simulink subsystem "Controls"  (R2024b)
settings: Solver=VariableStepAuto  StartTime=0.0  StopTime=10.0  RelTol=1e-3
undefined symbols (not defined in the file): D1, DiscIntNeverNeededParam, lag, Tctrl, test_alpha, Ts, Yg
libraries: powerlib_extras x74, simulink x10
(part 2 of 7)

== system Controls/fault_trigger ==
  pulse : Inport
  set : Inport  Port=2
  Compare To Constant{1..4,6..7} (6 alike) : simulink/Logic and Bit Operations/Compare To Constant  relop=>=  const=0.5  OutDataTypeStr=uint8  ZeroCross=off
  Constant : Constant  Value=[0 0]
  Demux1 : Demux  Outputs=[7 1 7]
  Demux2 : Demux  Outputs=[1 3 3]
  Demux4 : Demux  Outputs=7
  Mux9 : Mux  Inputs=8
  Product{1..4,6..10} (9 alike) : Product  RndMeth=Zero
  Terminator : Terminator
  faultgen : Subsystem
  DCtrig : Outport
  fault : Outport  Port=2
  wires:
  faultgen/3(trig) -> DCtrig/1  "trigger sig"
  pulse/1 -> faultgen/5(pulse)
  faultgen/1(fault) -> Product9/2, Product8/2, Product7/2, Product4/2, Product3/2, Product2/2, Product1/2
  Constant/1 -> faultgen/4(pert_set)
  Demux2/2 -> faultgen/2(Tst_set)
  Demux2/1 -> faultgen/1(Tacq)
  Demux2/3 -> faultgen/3(Tdr_set)
  faultgen/2(pertb) -> Terminator/1
  Demux1/2 -> Mux9/8
  Demux1/1 -> Demux4/1
  set/1 -> Demux1/1
  Mux9/1 -> fault/1
  Product9/1 -> Product10/1
  Product10/1 -> Mux9/7  "inv_fault"
  Demux4/7 -> Product10/2, Compare To Constant7/1
  Compare To Constant7/1 -> Product9/1
  Demux4/6 -> Product6/2, Compare To Constant6/1
  Demux4/5 -> Product7/1
  Demux4/4 -> Compare To Constant4/1
  Demux4/3 -> Compare To Constant3/1
  Demux4/2 -> Compare To Constant2/1
  Demux4/1 -> Compare To Constant1/1
  Demux1/3 -> Demux2/1
  Product8/1 -> Product6/1
  Compare To Constant6/1 -> Product8/1
  Product7/1 -> Mux9/6  "Fault_ac"
  Product4/1 -> Mux9/4  "Fault_dc"
  Compare To Constant4/1 -> Product4/1
  Product3/1 -> Mux9/3  "gammastep"
  Compare To Constant3/1 -> Product3/1
  Product2/1 -> Mux9/2  "Vdstep"
  Compare To Constant2/1 -> Product2/1
  Product1/1 -> Mux9/1  "Idrefstep"
  Compare To Constant1/1 -> Product1/1
  Product6/1 -> Mux9/5  "rect_fault"

== system Controls/paraconv ==
  In1 : Inport
  Demux : Demux  Outputs=[2 2 2 ]
  Kp/Ki-Ki to Kp Ki1 : Subsystem
  Kp/Ki-Ki to Kp Ki2 : Subsystem
  Kp/Ki-Ki to Kp Ki3 : Subsystem
  Mux2 : Mux  Inputs=3
  Out1 : Outport
  wires:
  Demux/3 -> Kp/Ki-Ki to Kp Ki3/1(i)
  Demux/2 -> Kp/Ki-Ki to Kp Ki2/1(i)  "KinvG"
  Demux/1 -> Kp/Ki-Ki to Kp Ki1/1(i)  "KinvV"
  In1/1 -> Demux/1
  Mux2/1 -> Out1/1
  Kp/Ki-Ki to Kp Ki3/1(o) -> Mux2/3
  Kp/Ki-Ki to Kp Ki2/1(o) -> Mux2/2
  Kp/Ki-Ki to Kp Ki1/1(o) -> Mux2/1

== system Controls/Master Control/Informations ==
  note: At start-up, both converters are deblocked and ramped up to the minimum current allowed in steady-state
      | with an adjustable rate  and application time in the "Start/Stop & Ramping Unit" subsystem. After the
      | system stabilisation the current is ramped up to its final value  with an adjustable rate and execution time.
      | Before stopping the converters the current is ramped down to the minimum reference.
  note: DESCRIPTION
  note: The rectifier and inverter current reference are generated in the master control. The reference
      | should be equal in both converters to avoid the loss of the margin. The converter starting and stopping is
      | initiated and the current reference can be ramped up or down.  A current step can be added to the
      | current reference for testing purpose.
  note: INTRODUCTION
  note: Master Control
  note: For testing purpose,  a step can be activated and added to the reference current at both
      | converters.

== system Controls/Master Control/Start//Stop ==
  note: Ramping
      | (modified from SPS demo)
  note: Start/Stop & Ramping
  note: Start/Stop sequence
  start : Inport
  Discrete Bistable : powerlib_extras/Discrete  Control Blocks/Discrete Bistable  Priority=488689760  SPSpriority=Set  ic=0  Ts=dt
  Discrete Edge Detector1 : powerlib_extras/Discrete  Control Blocks/Discrete Edge Detector  model=Rising  ic=0  Ts=dt
  Discrete Edge Detector2 : powerlib_extras/Discrete  Control Blocks/Discrete Edge Detector  model=Rising  ic=0  Ts=dt
  Logical Operator1 : Logic  Operator=NOT  AllPortsSameDT=off
  Logical Operator3 : Logic  AllPortsSameDT=off
  Minimum ref : Constant  Value=Min_ref
  Relational Operator1 : RelationalOperator  Operator=<=  InputSameDT=off
  S1 : Subsystem  mask(RAMPING UNIT){Min_ref=Min_ref, SS_ramp=SS_ramp, F_up=F_up, up_slope=up_slope, T_up=T_up, F_down=F_down, down_slope=down_slope, T_down=T_down}
      mask prompts: Min_ref "Minimum Value (pu):"; SS_ramp "Start-Stop ramp (pu/s):"; F_up "Final Up Value (pu):"; up_slope "Up Slope (pu/s):"; T_up "Ramping Up Time (s):"; F_down "Final Down Value (pu):"; down_slope "Down Slope (pu/s):"; T_down "Ramping Down Time (s):"
      mask init:
      | T_up_final      =  T_up + (F_up - Min_ref)/up_slope;
      | T_down_final =   T_down + (F_down-F_up)/down_slope;
      | T_ramp  = [0, T_up, T_up_final,  T_down,  T_down_final, 9999]';
      | U_ramp = [0, 0, F_up-Min_ref,  F_up-Min_ref,  F_down- Min_ref,  F_down - Min_ref]';
      mask Display: disp('Ramping\n Unit')
  Unit Delay : UnitDelay  SampleTime=dt  HasFrameUpgradeWarning=on
  Id_ref_ramp : Outport
  "Stop " : Outport  Port=2
  wires:
  Logical Operator1/1 -> Logical Operator3/2
  start/1 -> Logical Operator1/1, S1/1(Start), Discrete Edge Detector1/1
  Discrete Edge Detector1/1 -> Discrete Bistable/1
  Relational Operator1/1 -> Logical Operator3/1
  Logical Operator3/1 -> Discrete Edge Detector2/1
  Unit Delay/1 -> Relational Operator1/1
  Minimum ref/1 -> Relational Operator1/2
  Discrete Bistable/2 -> "Stop "/1
  S1/1(Out1) -> Id_ref_ramp/1, Unit Delay/1
  Discrete Edge Detector2/1 -> Discrete Bistable/2

== system Controls/Pole 1 Inverter Control and Protection/12-pulse Firing Control ==
  alpha_ord (deg) : Inport
  Vabc (pu) : Inport  Port=2
  Block : Inport  Port=3
  Data Type Conversion : DataTypeConversion  OutDataTypeStr=double
  Mux1 : Mux  Inputs=6
  PLL : Subsystem
  Freq : Outport
  fpu_I : Outport  Port=2
  wires:
  PLL/3(Vc) -> Mux1/4
  PLL/2(Vb) -> Mux1/3
  PLL/1(Va) -> Mux1/2
  Mux1/1 -> fpu_I/1
  Data Type Conversion/1 -> Mux1/6
  Block/1 -> Data Type Conversion/1
  alpha_ord (deg)/1 -> Mux1/1
  PLL/4(Freq) -> Mux1/5, Freq/1
  Vabc (pu)/1 -> PLL/1(Vabc(pu))

== system Controls/Pole 1 Inverter Control and Protection/Gamma Measurement ==
  note: PU scaling is made
      | in the SS_
  note: PU scaling is made
      | in the SS_
  Vabc : Inport
  Freq : Inport  Port=2
  IthyY : Inport  Port=3
  IthyD : Inport  Port=4
  Discrete Gamma Measurement (D bridge) : powerlib_extras/Discrete  Control Blocks/Discrete Gamma Measurement  transfo_type=Yg / D1(lag)  f0=50  Ith_min=0.001  Interpolation=off  V_tol=0.01  Ts=Tctrl
  Discrete Gamma Measurement (Y bridge) : powerlib_extras/Discrete  Control Blocks/Discrete Gamma Measurement  transfo_type=Yg / Y  f0=50  Ith_min=0.001  Interpolation=off  V_tol=0.01  Ts=Tctrl
  MinMax1 : MinMax  Inputs=2  InputSameDT=on  SaturateOnIntegerOverflow=on
  Selector : Selector  InputPortWidth=6  IndexOptions=Index vector (dialog)  Indices=1  OutputSizes=1
  Selector1 : Selector  InputPortWidth=6  IndexOptions=Index vector (dialog)  Indices=1  OutputSizes=1
  Sum1 : Sum  InputSameDT=on  SaturateOnIntegerOverflow=on  OutDataTypeStr=Inherit: Same as first input
  Terminator2 : Terminator
  k : Gain  Gain=0.5  SaturateOnIntegerOverflow=on  OutDataTypeStr=Inherit: Same as input  ParamDataTypeStr=Inherit: Same as input
  gama_min : Outport
  gama_mean : Outport  Port=2
  ISw1Y_pu : Outport  Port=3
  Ucom1Y_pu : Outport  Port=4
  wires:
  [Ucom1Y_pu] -> Ucom1Y_pu/1
  [ISw1Y_pu] -> ISw1Y_pu/1
  IthyY/1 -> Discrete Gamma Measurement (Y bridge)/1, Selector1/1
  IthyD/1 -> Discrete Gamma Measurement (D bridge)/1
  Freq/1 -> Discrete Gamma Measurement (D bridge)/3, Discrete Gamma Measurement (Y bridge)/3
  Selector1/1 -> [ISw1Y_pu]
  Selector/1 -> [Ucom1Y_pu]
  k/1 -> gama_mean/1
  Sum1/1 -> k/1
  MinMax1/1 -> gama_min/1
  Discrete Gamma Measurement (D bridge)/1 -> MinMax1/2  "gamma min D"
  Discrete Gamma Measurement (D bridge)/2 -> Sum1/2
  Discrete Gamma Measurement (D bridge)/3 -> Terminator2/1
  Discrete Gamma Measurement (Y bridge)/2 -> Sum1/1
  Discrete Gamma Measurement (Y bridge)/3 -> Selector/1
  Discrete Gamma Measurement (Y bridge)/1 -> MinMax1/1  "gamma min Y"
  Vabc/1 -> Discrete Gamma Measurement (D bridge)/2, Discrete Gamma Measurement (Y bridge)/2

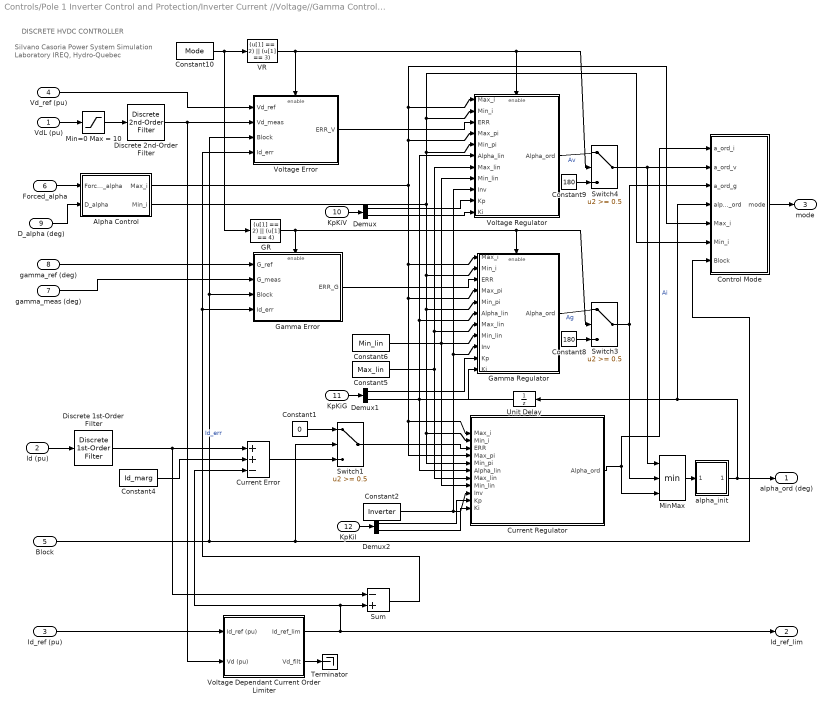
== system Controls/Pole 1 Inverter Control and Protection/Inverter Current //Voltage//Gamma Controller  ==
  note: Silvano Casoria
      | Power System Simulation Laboratory
      |  IREQ, Hydro-Quebec
  note: DISCRETE HVDC CONTROLLER
  VdL (pu) : Inport
  Id (pu) : Inport  Port=2
  Id_ref (pu) : Inport  Port=3
  Vd_ref (pu) : Inport  Port=4
  Block : Inport  Port=5
  Forced_alpha : Inport  Port=6
  gamma_meas (deg) : Inport  Port=7
  gamma_ref (deg) : Inport  Port=8
  D_alpha (deg) : Inport  Port=9
  KpKiV : Inport  Port=10
  KpKiG : Inport  Port=11
  KpKiI : Inport  Port=12
  Alpha Control : Subsystem
  Constant1 : Constant  Value=0
  Constant10 : Constant  Value=Mode
  Constant2 : Constant  Value=Inverter
  Constant4 : Constant  Value=Id_marg
  Constant5 : Constant  Value=Max_lin
  Constant6 : Constant  Value=Min_lin
  Constant8 : Constant  Value=180
  Constant9 : Constant  Value=180
  "Control Mode " : Subsystem
  Current Error : Sum  Inputs=++-  InputSameDT=on  SaturateOnIntegerOverflow=on  OutDataTypeStr=Inherit: Same as first input
  Current Regulator : Subsystem  mask(PI Regulator  With  External  Limits (Discrete)){Kp=Kp_I, Ki=Ki_I, IC_i=ICi_I, On_lin=on, dt=dt}
      mask prompts: Kp "Kp (deg/pu):"; Ki "Ki (deg/pu/s):"; IC_i "Integrator Initial Condition (deg):"; On_lin "Linearization  (On)"; dt "Sample time (s):"
      mask help: For the linearization it is important to specifie the mode of operation i.e. rectifier or inverter (negation of rectifier).
      mask Display: disp('PI Regulator\nWith external limits\n(Linearized Kp)\n(Discrete)\n\n')
  Demux : Demux  Outputs=2
  Demux1 : Demux  Outputs=2
  Demux2 : Demux  Outputs=2
  Discrete 1st-Order Filter : powerlib_extras/Discrete  Control Blocks/Discrete 1st-Order Filter  FilterType=Lowpass  Tc=T_I  Ts=dt  Initialize=off  Vac_Init=[0.8 -25 60]  Vdc_Init=-0.4  PlotResponse=off  param1=[1 500 0.1]
  Discrete 2nd-Order Filter : powerlib_extras/Discrete  Control Blocks/Discrete  2nd-Order Filter  FilterType=Lowpass  Fo=f0_V  Zeta=Z_V  Ts=dt  Initialize=off  Vac_Init=[0.8 -25 60]  Vdc_Init=-0.4  PlotResponse=off  param1=[1 500 1]
  GR : Fcn  Expr=(u[1] == 2) || (u[1] == 4)
  Gamma Error : Subsystem  TreatAsAtomicUnit=on
  Gamma Regulator : Subsystem  TreatAsAtomicUnit=on
  Min=0 Max = 10 : Saturate  UpperLimit=10  LowerLimit=0
  MinMax : MinMax  Inputs=3  InputSameDT=on  SaturateOnIntegerOverflow=on
  Sum : Sum  Inputs=-+  InputSameDT=on  SaturateOnIntegerOverflow=on  OutDataTypeStr=Inherit: Same as first input
  Switch1 : Switch  Threshold=0.5
  Switch3 : Switch  Threshold=0.5
  Switch4 : Switch  Threshold=0.5
  Terminator : Terminator
  Unit Delay : UnitDelay  SampleTime=dt  HasFrameUpgradeWarning=on
  VR : Fcn  Expr=(u[1] == 2) || (u[1] == 3)
  Voltage Dependant Current Order Limiter : Subsystem  mask(Voltage Dependent Current Order Limiter  (Discrete)){Vd_seuil=Vd_seuil, Vd_min=Vd_min, Id_min=Id_min, Id_min_abs=Id_min_abs, Tu=Tup, pas=dt}
      mask prompts: Vd_seuil "Vd seuil (pu):"; Vd_min "Vd min (pu):"; Id_min "Id min (pu):"; Id_min_abs "Id min abs (pu):"; Tu "Up Time constant (s):"; pas "Sample time (s):"
      mask Display: disp('VDCOL\n (Discrete)')
  Voltage Error : Subsystem  TreatAsAtomicUnit=on
  Voltage Regulator : Subsystem  TreatAsAtomicUnit=on
  alpha_init : Subsystem
  alpha_ord (deg) : Outport
  Id_ref_lim : Outport  Port=2
  mode : Outport  Port=3
  wires:
  Demux2/1 -> Current Regulator/10(Kp)
  Demux2/2 -> Current Regulator/11(Ki)
  KpKiI/1 -> Demux2/1
  Demux1/1 -> Gamma Regulator/10(Kp)
  Demux1/2 -> Gamma Regulator/11(Ki)
  KpKiG/1 -> Demux1/1
  Demux/1 -> Voltage Regulator/10(Kp)
  Demux/2 -> Voltage Regulator/11(Ki)
  KpKiV/1 -> Demux/1
  Forced_alpha/1 -> Alpha Control/1(Forced_alpha)
  "Control Mode "/1(mode) -> mode/1
  Voltage Error/1(ERR_V) -> Voltage Regulator/3(ERR)
  Vd_ref (pu)/1 -> Voltage Error/1(Vd_ref)
  Sum/1 -> Gamma Error/4(Id_err), Voltage Error/4(Id_err)  "Id_err"
  gamma_meas (deg)/1 -> Gamma Error/2(G_meas)
  gamma_ref (deg)/1 -> Gamma Error/1(G_ref)
  Gamma Error/1(ERR_G) -> Gamma Regulator/3(ERR)
  Constant1/1 -> Switch1/1
  Switch4/1 -> "Control Mode "/2(a_ord_v), MinMax/1
  Switch3/1 -> "Control Mode "/3(a_ord_g), MinMax/2
  Current Regulator/1(Alpha_ord) -> "Control Mode "/1("a_ord_i "), MinMax/3  "Ai"
  Constant9/1 -> Switch4/3
  Voltage Regulator/1(Alpha_ord) -> Switch4/1  "Av"
  Constant8/1 -> Switch3/3
  Gamma Regulator/1(Alpha_ord) -> Switch3/1  "Ag"
  Switch1/1 -> Current Regulator/3(ERR)
  Constant2/1 -> Current Regulator/9(Inv), Gamma Regulator/9(Inv), Voltage Regulator/9(Inv)
  Block/1 -> Voltage Error/3(Block), Gamma Error/3(Block), "Control Mode "/7(Block), Switch1/2
  Alpha Control/2(Min_i) -> Voltage Regulator/5(Min_pi), "Control Mode "/6(Min_i), Voltage Regulator/2(Min_i), Gamma Regulator/2(Min_i), Gamma Regulator/5(Min_pi), Current Regulator/2(Min_i), Current Regulator/5(Min_pi)
  Constant5/1 -> Current Regulator/7(Max_lin), Voltage Regulator/7(Max_lin), Gamma Regulator/7(Max_lin)
  alpha_init/1(Out1) -> "Control Mode "/4(alpha_ord), Unit Delay/1, alpha_ord (deg)/1
  Unit Delay/1 -> Current Regulator/6(Alpha_lin), Voltage Regulator/6(Alpha_lin), Gamma Regulator/6(Alpha_lin)
  MinMax/1 -> alpha_init/1(In1)
  Current Error/1 -> Switch1/3
  Discrete 1st-Order Filter/1 -> Current Error/1, Sum/1
  Id (pu)/1 -> Discrete 1st-Order Filter/1
  VdL (pu)/1 -> Min=0 Max = 10/1
  Min=0 Max = 10/1 -> Discrete 2nd-Order Filter/1
  Discrete 2nd-Order Filter/1 -> Voltage Error/2(Vd_meas), Voltage Dependant Current Order Limiter/2(Vd (pu))
  Voltage Dependant Current Order Limiter/1(Id_ref_lim) -> Current Error/3, Sum/2, Id_ref_lim/1
  Voltage Dependant Current Order Limiter/2(Vd_filt) -> Terminator/1
  Id_ref (pu)/1 -> Voltage Dependant Current Order Limiter/1(Id_ref (pu))
  Constant4/1 -> Current Error/2
  Constant6/1 -> Current Regulator/8(Min_lin), Voltage Regulator/8(Min_lin), Gamma Regulator/8(Min_lin)
  Alpha Control/1(Max_i) -> Voltage Regulator/4(Max_pi), "Control Mode "/5(Max_i), Voltage Regulator/1(Max_i), Gamma Regulator/1(Max_i), Gamma Regulator/4(Max_pi), Current Regulator/1(Max_i), Current Regulator/4(Max_pi)
  D_alpha (deg)/1 -> Alpha Control/2(D_alpha)
  VR/1 -> Voltage Regulator/Enable, Switch4/2, Voltage Error/Enable
  Constant10/1 -> GR/1, VR/1
  GR/1 -> Gamma Regulator/Enable, Switch3/2, Gamma Error/Enable

== system Controls/Pole 1 Inverter Control and Protection/Inverter Protections ==
  Uabc (pu) : Inport
  1st-Order T=3.3 ms : powerlib_extras/Discrete  Control Blocks/Discrete 1st-Order Filter  FilterType=Lowpass  Tc=0.0033  Ts=Tctrl  Initialize=off  Vac_Init=[0.8 -25 60]  Vdc_Init=-0.4  PlotResponse=off  param1=[1 500 0.1]
  Commutation Failure Prevention Control (CFPREV) : Subsystem  mask(Commutation Failure Prevention Control){STATE=on, T_ss=0.64, ab_level=0.1, ab_gain=25, z_level=0.1, z_gain=25, fn=60, Filter=[2.0, 1.0], Ts=Tctrl}
      mask prompts: STATE "ON State"; T_ss "Simulation Steady_State Time (s):"; ab_level "ab level (pu):"; ab_gain "ab gain (deg/pu):"; z_level "z level (pu):"; z_gain "z gain (deg/pu):"; fn "Base frequency (Hz):"; Filter "Filter Time const. and Iinitial condition [T(s), Ic (pu)]:"; Ts "Sample Time (s):"
      mask help:
      | The protective function, used in the inverter, mitigates commutation failures due to AC voltage dips. After a fault detection (three-phase or one-phase) an angle value (AMIN_CFPREV) is sent to the converter control in order to be deducted from the maximum delay angle limit (alpha_max). Practicaly, the commutation margin is consequently enlarged reducing therfore the risk of commutation failures.
      |
      |      The CLARK transformation is used for three-phase fault  detection and the zero-sequence voltage evaluation. The detection is based  on instantaneous values, which ensure fast reaction of the control system when AC faults occurs.
      |
      |      Press Help to get the reference with the  detailed description of the function and  parameters.
      |
      | Note: To accelerate the function initialisation, the first parameter (Simulation Steady_State Time) is used. It corresponds to the time when the input voltages reache  the steady-state value.
      mask init:
      | T_periode = 0.6/fn;    % More then half the period
      | filt_tc = Filter(1);
      | filt_ic = Filter(2);
      | 
      | if (STATE)
      | 	str = 'ON';
      | else
      | 	str = 'OFF';
      | end
      mask Help:
      | Ref. "A Novel Method to Mitigate Commutation Failures in HVDC Systems,"
      | Lidong Zhang, Lars Dofnas ABB Utilities Power System Technology,
      | Proceedings PowerCon 2002, Volume: 1 , 13-17 Oct. 2002,  Page(s): 51-56 vol.1.
      mask Display: disp(['\n\n\n State:[',str,']'])
  Informations : Subsystem
      mask Display: disp('?')
  Low AC Voltage Detection (LACVD) : Subsystem  TreatAsAtomicUnit=on  mask(Low AC voltage detection){STATE=on, Ref_1=0.75, dt=Ts}
      mask prompts: STATE "ON State"; Ref_1 "Detection level (pu):"; dt "Sample time (s):"
      mask help:
      | This bloc detects a low AC voltage condition on the commutation busbar and is used in the DC protection scheme. Its purpose is to descriminate between a drop in the AC voltage caused by a fault on the DC line or by a fault on the AC side.
      |
      |      An AC fault detection (Low_ac_voltage output signal) will occur when the AC voltage input (recified three-phase AC voltage) drops below a certain reference value (Detection
      | level).
      |
      |      In order to minimize the simulation time, an enabled susbystem having a sample time of 1 (ms) has been used in accordance with an acceptable precision.
      mask init:
      | if (STATE)
      | 	str = 'ON';
      | else
      | 	str = 'OFF';
      | end
      mask Display: disp(['\n\n\n\nState:[',str,']'])
  Udio_6p : Subsystem
  Low_AC_Voltage : Outport
  AMIN_CFPREV : Outport  Port=2
  wires:
  Commutation Failure Prevention Control (CFPREV)/1(AMIN_CFPREV (deg)) -> AMIN_CFPREV/1
  Low AC Voltage Detection (LACVD)/1(Low_AC_Voltage) -> Low_AC_Voltage/1
  Uabc (pu)/1 -> Udio_6p/1(Uabc (pu)), Commutation Failure Prevention Control (CFPREV)/1(Uabc (pu))
  Udio_6p/1(Udio_6p) -> 1st-Order T=3.3 ms/1
  1st-Order T=3.3 ms/1 -> Low AC Voltage Detection (LACVD)/1(Uac (pu))

== system Controls/Pole 1 Inverter Control and Protection/Polarity_check ==
  converter_position : Inport
  Vdc_line : Inport  Port=2
  Vdc_neutral : Inport  Port=3
  Idc_in : Inport  Port=4
  Add : Sum  Inputs=+-
  Constant : Constant
  Constant1 : Constant  Value=-1
  Constant2 : Constant  Value=3
  Discrete 1st-Order Filter : powerlib_extras/Discrete  Control Blocks/Discrete 1st-Order Filter  FilterType=Lowpass  Tc=5  Ts=Tctrl  Initialize=off  Vac_Init=[0.8 -25 60]  Vdc_Init=-0.4  PlotResponse=off  param1=[1 500 0.1]
  MinMax : MinMax  Function=max  SampleTime=Tctrl
  Multiport Switch : MultiPortSwitch  DataPortOrder=Zero-based contiguous  Inputs=2  zeroidx=on  SaturateOnIntegerOverflow=off  InputSameDT=off
  Mux : Mux  Inputs=2
  Product : Product  RndMeth=Zero
  Product1 : Product  RndMeth=Zero
  Product2 : Product  RndMeth=Zero
  Relational Operator : RelationalOperator  OutDataTypeStr=boolean  InputSameDT=off
  Vdc_meas : Outport
  Idc_meas : Outport  Port=2
  wires:
  Product2/1 -> Idc_meas/1
  Relational Operator/1 -> Multiport Switch/1
  Constant2/1 -> Relational Operator/2
  converter_position/1 -> Relational Operator/1
  Idc_in/1 -> Product2/2
  Multiport Switch/1 -> Product2/1, Product1/1, Product/1
  Constant1/1 -> Multiport Switch/3
  Constant/1 -> Multiport Switch/2
  Vdc_neutral/1 -> Product1/2
  Product1/1 -> Discrete 1st-Order Filter/1
  Product/1 -> Mux/1, Add/1
  Vdc_line/1 -> Product/2
  MinMax/1 -> Vdc_meas/1
  Mux/1 -> MinMax/1
  Add/1 -> Mux/2
  Discrete 1st-Order Filter/1 -> Add/2

== system Controls/Pole 1 Inverter Control and Protection/Ref_and_step_ctrl ==
  Vd_step : Inport
  Gamma_step : Inport  Port=2
  Add : Sum
  Add1 : Sum
  Discrete Monostable1 : powerlib_extras/Discrete  Control Blocks/Discrete Monostable  EdgeDetect=Rising  t_mono=0.2  ic=0  Ts=Tctrl
  Discrete Monostable2 : powerlib_extras/Discrete  Control Blocks/Discrete Monostable  EdgeDetect=Rising  t_mono=0.1  ic=0  Ts=Tctrl
  Gamma min : Constant  Value=18
  Vd_ref : Constant  Value=1.0
  g : Gain  Gain=5  SaturateOnIntegerOverflow=on  OutDataTypeStr=Inherit: Same as input  ParamDataTypeStr=Inherit: Same as input
  g1 : Gain  Gain=-0.1  SaturateOnIntegerOverflow=on  OutDataTypeStr=Inherit: Same as input  ParamDataTypeStr=Inherit: Same as input
  Vd_ref_out : Outport
  Gamma_ref_out : Outport  Port=2
  wires:
  Add/1 -> Gamma_ref_out/1
  Gamma_step/1 -> Discrete Monostable1/1
  Discrete Monostable1/1 -> g/1
  Gamma min/1 -> Add/2
  g/1 -> Add/1
  Vd_step/1 -> Discrete Monostable2/1
  Add1/1 -> Vd_ref_out/1
  g1/1 -> Add1/1
  Discrete Monostable2/1 -> g1/1
  Vd_ref/1 -> Add1/2

== system Controls/Pole 1 Rectifier Control and Protection/12-pulse Firing Control ==
  alpha_ord (deg) : Inport
  Vabc (pu) : Inport  Port=2
  Block : Inport  Port=3
  Data Type Conversion : DataTypeConversion  OutDataTypeStr=double
  Mux2 : Mux  Inputs=6
  PLL : Subsystem
  Freq : Outport
  fpuR : Outport  Port=2
  wires:
  Data Type Conversion/1 -> Mux2/6
  Mux2/1 -> fpuR/1
  Block/1 -> Data Type Conversion/1
  alpha_ord (deg)/1 -> Mux2/1
  PLL/4(Freq) -> Mux2/5, Freq/1
  PLL/3(Vc) -> Mux2/4
  PLL/2(Vb) -> Mux2/3
  PLL/1(Va) -> Mux2/2
  Vabc (pu)/1 -> PLL/1(Vabc(pu))

== system Controls/Pole 1 Rectifier Control and Protection/Polarity_check ==
  converter_position : Inport
  Vdc_line : Inport  Port=2
  Vdc_neutral : Inport  Port=3
  Idc_in : Inport  Port=4
  Add : Sum  Inputs=+-
  Constant : Constant
  Constant1 : Constant  Value=-1
  Constant2 : Constant  Value=3
  Discrete 1st-Order Filter : powerlib_extras/Discrete  Control Blocks/Discrete 1st-Order Filter  FilterType=Lowpass  Tc=5  Ts=Tctrl  Initialize=off  Vac_Init=[0.8 -25 60]  Vdc_Init=-0.4  PlotResponse=off  param1=[1 500 0.1]
  MinMax : MinMax  Function=max  SampleTime=Tctrl
  Multiport Switch : MultiPortSwitch  DataPortOrder=Zero-based contiguous  Inputs=2  zeroidx=on  SaturateOnIntegerOverflow=off  InputSameDT=off
  Mux : Mux  Inputs=2
  Product : Product  RndMeth=Zero
  Product1 : Product  RndMeth=Zero
  Product2 : Product  RndMeth=Zero
  Relational Operator : RelationalOperator  OutDataTypeStr=boolean  InputSameDT=off
  Vdc_meas : Outport
  Idc_meas : Outport  Port=2
  wires:
  Product2/1 -> Idc_meas/1
  Relational Operator/1 -> Multiport Switch/1
  Constant2/1 -> Relational Operator/2
  converter_position/1 -> Relational Operator/1
  Idc_in/1 -> Product2/2
  Multiport Switch/1 -> Product2/1, Product1/1, Product/1
  Constant1/1 -> Multiport Switch/3
  Constant/1 -> Multiport Switch/2
  Vdc_neutral/1 -> Product1/2
  Product1/1 -> Discrete 1st-Order Filter/1
  Product/1 -> Mux/1, Add/1
  Vdc_line/1 -> Product/2
  MinMax/1 -> Vdc_meas/1
  Mux/1 -> MinMax/1
  Add/1 -> Mux/2
  Discrete 1st-Order Filter/1 -> Add/2

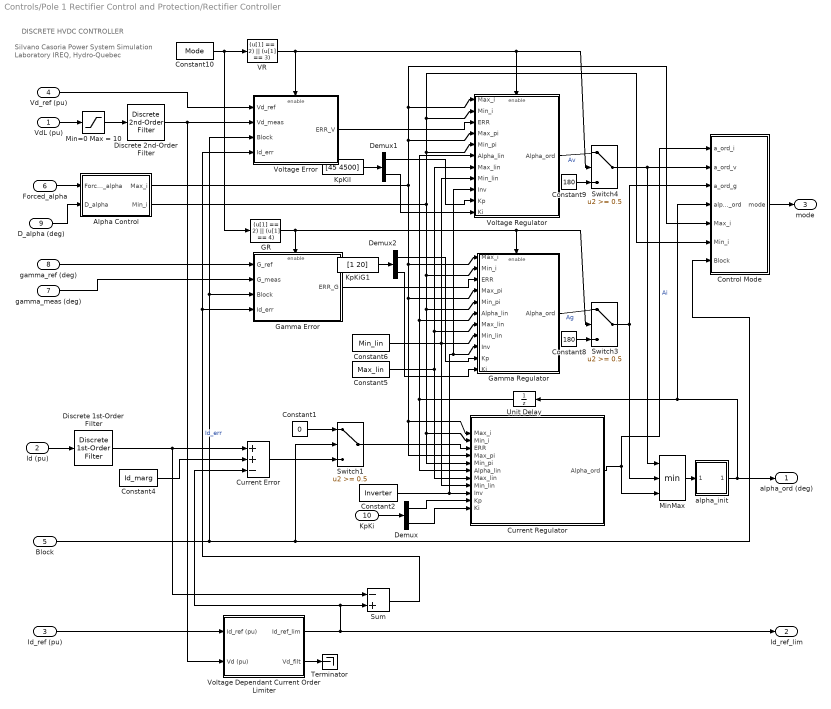
== system Controls/Pole 1 Rectifier Control and Protection/Rectifier Controller ==
  note: Silvano Casoria
      | Power System Simulation Laboratory
      |  IREQ, Hydro-Quebec
  note: DISCRETE HVDC CONTROLLER
  VdL (pu) : Inport
  Id (pu) : Inport  Port=2
  Id_ref (pu) : Inport  Port=3
  Vd_ref (pu) : Inport  Port=4
  Block : Inport  Port=5
  Forced_alpha : Inport  Port=6
  gamma_meas (deg) : Inport  Port=7
  gamma_ref (deg) : Inport  Port=8
  D_alpha (deg) : Inport  Port=9
  KpKi : Inport  Port=10
  Alpha Control : Subsystem
  Constant1 : Constant  Value=0
  Constant10 : Constant  Value=Mode
  Constant2 : Constant  Value=Inverter
  Constant4 : Constant  Value=Id_marg
  Constant5 : Constant  Value=Max_lin
  Constant6 : Constant  Value=Min_lin
  Constant8 : Constant  Value=180
  Constant9 : Constant  Value=180
  "Control Mode " : Subsystem
  Current Error : Sum  Inputs=++-  InputSameDT=on  SaturateOnIntegerOverflow=on  OutDataTypeStr=Inherit: Same as first input
  Current Regulator : Subsystem  mask(PI Regulator  With  External  Limits (Discrete)){Kp=Kp_I, Ki=Ki_I, IC_i=ICi_I, On_lin=on, dt=dt}
      mask prompts: Kp "Kp (deg/pu):"; Ki "Ki (deg/pu/s):"; IC_i "Integrator Initial Condition (deg):"; On_lin "Linearization  (On)"; dt "Sample time (s):"
      mask help: For the linearization it is important to specifie the mode of operation i.e. rectifier or inverter (negation of rectifier).
      mask Display: disp('PI Regulator\nWith external limits\n(Linearized Kp)\n(Discrete)\n\n')
  Demux : Demux  Outputs=2
  Demux1 : Demux  Outputs=2
  Demux2 : Demux  Outputs=2
  Discrete 1st-Order Filter : powerlib_extras/Discrete  Control Blocks/Discrete 1st-Order Filter  FilterType=Lowpass  Tc=T_I  Ts=dt  Initialize=off  Vac_Init=[0.8 -25 60]  Vdc_Init=-0.4  PlotResponse=off  param1=[1 500 0.1]
  Discrete 2nd-Order Filter : powerlib_extras/Discrete  Control Blocks/Discrete  2nd-Order Filter  FilterType=Lowpass  Fo=f0_V  Zeta=Z_V  Ts=dt  Initialize=off  Vac_Init=[0.8 -25 60]  Vdc_Init=-0.4  PlotResponse=off  param1=[1 500 1]
  GR : Fcn  Expr=(u[1] == 2) || (u[1] == 4)
  Gamma Error : Subsystem  TreatAsAtomicUnit=on
  Gamma Regulator : Subsystem  TreatAsAtomicUnit=on
  KpKiG1 : Constant  Value=[1 20]  OutDataTypeStr=double
  KpKiI : Constant  Value=[45 4500]
  Min=0 Max = 10 : Saturate  UpperLimit=10  LowerLimit=0
  MinMax : MinMax  Inputs=3  InputSameDT=on  SaturateOnIntegerOverflow=on
  Sum : Sum  Inputs=-+  InputSameDT=on  SaturateOnIntegerOverflow=on  OutDataTypeStr=Inherit: Same as first input
  Switch1 : Switch  Threshold=0.5
  Switch3 : Switch  Threshold=0.5
  Switch4 : Switch  Threshold=0.5
  Terminator : Terminator
  Unit Delay : UnitDelay  SampleTime=dt  HasFrameUpgradeWarning=on
  VR : Fcn  Expr=(u[1] == 2) || (u[1] == 3)
  Voltage Dependant Current Order Limiter : Subsystem  mask(Voltage Dependent Current Order Limiter  (Discrete)){Vd_seuil=Vd_seuil, Vd_min=Vd_min, Id_min=Id_min, Id_min_abs=Id_min_abs, Tu=Tup, pas=dt}
      mask prompts: Vd_seuil "Vd seuil (pu):"; Vd_min "Vd min (pu):"; Id_min "Id min (pu):"; Id_min_abs "Id min abs (pu):"; Tu "Up Time constant (s):"; pas "Sample time (s):"
      mask Display: disp('VDCOL\n (Discrete)')
  Voltage Error : Subsystem  TreatAsAtomicUnit=on
  Voltage Regulator : Subsystem  TreatAsAtomicUnit=on
  alpha_init : Subsystem
  alpha_ord (deg) : Outport
  Id_ref_lim : Outport  Port=2
  mode : Outport  Port=3
  wires:
  Demux/1 -> Current Regulator/10(Kp)
  Demux/2 -> Current Regulator/11(Ki)
  Demux2/1 -> Gamma Regulator/10(Kp)
  Demux2/2 -> Gamma Regulator/11(Ki)
  KpKiG1/1 -> Demux2/1
  Demux1/1 -> Voltage Regulator/10(Kp)
  Demux1/2 -> Voltage Regulator/11(Ki)
  KpKiI/1 -> Demux1/1
  KpKi/1 -> Demux/1
  Forced_alpha/1 -> Alpha Control/1(Forced_alpha)
  "Control Mode "/1(mode) -> mode/1
  Voltage Error/1(ERR_V) -> Voltage Regulator/3(ERR)
  Vd_ref (pu)/1 -> Voltage Error/1(Vd_ref)
  Sum/1 -> Gamma Error/4(Id_err), Voltage Error/4(Id_err)  "Id_err"
  gamma_meas (deg)/1 -> Gamma Error/2(G_meas)
  gamma_ref (deg)/1 -> Gamma Error/1(G_ref)
  Gamma Error/1(ERR_G) -> Gamma Regulator/3(ERR)
  Constant1/1 -> Switch1/1
  Switch4/1 -> "Control Mode "/2(a_ord_v), MinMax/1
  Switch3/1 -> "Control Mode "/3(a_ord_g), MinMax/2
  Current Regulator/1(Alpha_ord) -> "Control Mode "/1("a_ord_i "), MinMax/3  "Ai"
  Constant9/1 -> Switch4/3
  Voltage Regulator/1(Alpha_ord) -> Switch4/1  "Av"
  Constant8/1 -> Switch3/3
  Gamma Regulator/1(Alpha_ord) -> Switch3/1  "Ag"
  Switch1/1 -> Current Regulator/3(ERR)
  Constant2/1 -> Current Regulator/9(Inv), Gamma Regulator/9(Inv), Voltage Regulator/9(Inv)
  Block/1 -> Voltage Error/3(Block), Gamma Error/3(Block), "Control Mode "/7(Block), Switch1/2
  Alpha Control/2(Min_i) -> Voltage Regulator/5(Min_pi), "Control Mode "/6(Min_i), Voltage Regulator/2(Min_i), Gamma Regulator/2(Min_i), Gamma Regulator/5(Min_pi), Current Regulator/2(Min_i), Current Regulator/5(Min_pi)
  Constant5/1 -> Current Regulator/7(Max_lin), Voltage Regulator/7(Max_lin), Gamma Regulator/7(Max_lin)
  alpha_init/1(Out1) -> "Control Mode "/4(alpha_ord), Unit Delay/1, alpha_ord (deg)/1
  Unit Delay/1 -> Current Regulator/6(Alpha_lin), Voltage Regulator/6(Alpha_lin), Gamma Regulator/6(Alpha_lin)
  MinMax/1 -> alpha_init/1(In1)
  Current Error/1 -> Switch1/3
  Discrete 1st-Order Filter/1 -> Current Error/1, Sum/1
  Id (pu)/1 -> Discrete 1st-Order Filter/1
  VdL (pu)/1 -> Min=0 Max = 10/1
  Min=0 Max = 10/1 -> Discrete 2nd-Order Filter/1
  Discrete 2nd-Order Filter/1 -> Voltage Error/2(Vd_meas), Voltage Dependant Current Order Limiter/2(Vd (pu))
  Voltage Dependant Current Order Limiter/1(Id_ref_lim) -> Current Error/3, Sum/2, Id_ref_lim/1
  Voltage Dependant Current Order Limiter/2(Vd_filt) -> Terminator/1
  Id_ref (pu)/1 -> Voltage Dependant Current Order Limiter/1(Id_ref (pu))
  Constant4/1 -> Current Error/2
  Constant6/1 -> Current Regulator/8(Min_lin), Voltage Regulator/8(Min_lin), Gamma Regulator/8(Min_lin)
  Alpha Control/1(Max_i) -> Voltage Regulator/4(Max_pi), "Control Mode "/5(Max_i), Voltage Regulator/1(Max_i), Gamma Regulator/1(Max_i), Gamma Regulator/4(Max_pi), Current Regulator/1(Max_i), Current Regulator/4(Max_pi)
  D_alpha (deg)/1 -> Alpha Control/2(D_alpha)
  VR/1 -> Voltage Regulator/Enable, Switch4/2, Voltage Error/Enable
  Constant10/1 -> GR/1, VR/1
  GR/1 -> Gamma Regulator/Enable, Switch3/2, Gamma Error/Enable

== system Controls/Pole 1 Rectifier Control and Protection/Rectifier Protections ==
  note: DC Protections (in Rectifier)
  Uabc (pu) : Inport
  VdL (pu) : Inport  Port=2
  Deblocked : Inport  Port=3
  Low_ac_volt_oth : Inport  Port=4
  1st-Order T=3.3 ms : powerlib_extras/Discrete  Control Blocks/Discrete 1st-Order Filter  FilterType=Lowpass  Tc=0.0033  Ts=Tctrl  Initialize=off  Vac_Init=[0.8 -25 60]  Vdc_Init=-0.4  PlotResponse=off  param1=[1 500 0.1]
  DC Fault Protection (DCPROT) : Subsystem  mask(DC fault protection (in Rectifier)){STATE=on, Ref1=0.5, T1=0.070, T2=0.05, polarity=Positive, dt=Ts}
      mask prompts: STATE "ON State"; Ref1 "Detection level (pu):"; T1 "Detection delay (s):"; T2 "Forced alpha duration (s):"; polarity "Voltage polarity:"; dt "Sample time (s):"
      mask help:
      | The protection is active in the rectifier. It will detect a fault on the DC side and will force the delay angle into the inverter region in order to extinguish the fault current.
      |      The fault detection on the DC line is based on the drop in the line to ground voltage.
      |      The normal voltage polarity (+ or -) of the line is a parameter as well as the reference level (Detection level) of the fault detection.
      |      A delay time (Detection delay) is used in the detection to descriminate between a line fault and other disturbances resulting in a low DC voltage.
      |      A delay time (200 ms) is allowed, after the DC system start-up, before activating the detection logic to make sure that the normal operating DC voltage is established.
      |      Also, an external signal (Lock) generated by another protective function (e.g. Low AC voltage detection) will lock the detection for a minimum amount of time (set by an Off Delay bloc) in order to descriminate between any fault causing a low DC voltage.
      |      A detection will triger a Forced alpha during an ajustable interval (Forced alpha duration) sufficient to allow for deionization of the fault path prior to re-application of voltage.
      |
      |      In order to minimize the simulation time, an enabled susbystem having a sample time of  2 (ms) has been used in accordance with an acceptable precision.
      mask init:
      | if (polarity == 1)
      | 	sign = 1;
      | else
      | 	sign = -1;
      | end
      | 
      | if (STATE)
      | 	str = 'ON';
      | else
      | 	str = 'OFF';
      | end
      mask TypeOptions polarity: Positive | Negative
      mask Display: disp(['\n\n\n\nState:[',str,']'])
  Informations : Subsystem
      mask Display: disp('?')
  Logical Operator6 : Logic  Operator=OR
  Low AC Voltage Detection (LACVD) : Subsystem  TreatAsAtomicUnit=on  mask(Low AC voltage detection){STATE=on, Ref_1=0.70, dt=Ts}
      mask prompts: STATE "ON State"; Ref_1 "Detection level (pu):"; dt "Sample time (s):"
      mask help:
      | This bloc detects a low AC voltage condition on the commutation busbar and is used in the DC protection scheme. Its purpose is to descriminate between a drop in the AC voltage caused by a fault on the DC line or by a fault on the AC side.
      |
      |      An AC fault detection (Low_ac_voltage output signal) will occur when the AC voltage input (recified three-phase AC voltage) drops below a certain reference value (Detection level).
      |
      |      In order to minimize the simulation time, an enabled susbystem having a sample time of 1 (ms) has been used in accordance with an acceptable precision.
      mask init:
      | if (STATE)
      | 	str = 'ON';
      | else
      | 	str = 'OFF';
      | end
      mask Display: disp(['\n\n\n\nState:[',str,']'])
  Udio_6p : Subsystem
  Forced_alpha : Outport
  Low_ac_voltage : Outport  Port=2
  wires:
  Deblocked/1 -> DC Fault Protection (DCPROT)/2(Deblocked)
  VdL (pu)/1 -> DC Fault Protection (DCPROT)/1(VdL (pu))
  Logical Operator6/1 -> DC Fault Protection (DCPROT)/3(Lock)
  Low_ac_volt_oth/1 -> Logical Operator6/2
  DC Fault Protection (DCPROT)/1(Forced_alpha) -> Forced_alpha/1
  Low AC Voltage Detection (LACVD)/1(Low_AC_Voltage) -> Low_ac_voltage/1, Logical Operator6/1
  Uabc (pu)/1 -> Udio_6p/1(Uabc (pu))
  Udio_6p/1(Udio_6p) -> 1st-Order T=3.3 ms/1
  1st-Order T=3.3 ms/1 -> Low AC Voltage Detection (LACVD)/1(Uac (pu))

== system Controls/Pole 2 Inverter Control and Protection/12-pulse Firing Control ==
  alpha_ord (deg) : Inport
  Vabc (pu) : Inport  Port=2
  Block : Inport  Port=3
  Data Type Conversion : DataTypeConversion  OutDataTypeStr=double
  Mux1 : Mux  Inputs=6
  PLL : Subsystem
  Freq : Outport
  fpu_I : Outport  Port=2
  wires:
  PLL/3(Vc) -> Mux1/4
  PLL/2(Vb) -> Mux1/3
  PLL/1(Va) -> Mux1/2
  Mux1/1 -> fpu_I/1
  Data Type Conversion/1 -> Mux1/6
  Block/1 -> Data Type Conversion/1
  alpha_ord (deg)/1 -> Mux1/1
  PLL/4(Freq) -> Mux1/5, Freq/1
  Vabc (pu)/1 -> PLL/1(Vabc(pu))

== system Controls/Pole 2 Inverter Control and Protection/Gamma Measurement ==
  note: PU scaling is made
      | in the SS_
  note: PU scaling is made
      | in the SS_
  Vabc : Inport
  Freq : Inport  Port=2
  IthyY : Inport  Port=3
  IthyD : Inport  Port=4
  Discrete Gamma Measurement (D bridge) : powerlib_extras/Discrete  Control Blocks/Discrete Gamma Measurement  transfo_type=Yg / D1(lag)  f0=50  Ith_min=0.001  Interpolation=off  V_tol=0.01  Ts=Tctrl
  Discrete Gamma Measurement (Y bridge) : powerlib_extras/Discrete  Control Blocks/Discrete Gamma Measurement  transfo_type=Yg / Y  f0=50  Ith_min=0.001  Interpolation=off  V_tol=0.01  Ts=Tctrl
  MinMax1 : MinMax  Inputs=2  InputSameDT=on  SaturateOnIntegerOverflow=on
  Selector : Selector  InputPortWidth=6  IndexOptions=Index vector (dialog)  Indices=1  OutputSizes=1
  Selector1 : Selector  InputPortWidth=6  IndexOptions=Index vector (dialog)  Indices=1  OutputSizes=1
  Sum1 : Sum  InputSameDT=on  SaturateOnIntegerOverflow=on  OutDataTypeStr=Inherit: Same as first input
  Terminator2 : Terminator
  k : Gain  Gain=0.5  SaturateOnIntegerOverflow=on  OutDataTypeStr=Inherit: Same as input  ParamDataTypeStr=Inherit: Same as input
  gama_min : Outport
  gama_mean : Outport  Port=2
  ISw1Y_pu : Outport  Port=3
  Ucom1Y_pu : Outport  Port=4
  wires:
  [Ucom1Y_pu] -> Ucom1Y_pu/1
  [ISw1Y_pu] -> ISw1Y_pu/1
  IthyY/1 -> Discrete Gamma Measurement (Y bridge)/1, Selector1/1
  IthyD/1 -> Discrete Gamma Measurement (D bridge)/1
  Freq/1 -> Discrete Gamma Measurement (D bridge)/3, Discrete Gamma Measurement (Y bridge)/3
  Selector1/1 -> [ISw1Y_pu]
  Selector/1 -> [Ucom1Y_pu]
  k/1 -> gama_mean/1
  Sum1/1 -> k/1
  MinMax1/1 -> gama_min/1
  Discrete Gamma Measurement (D bridge)/1 -> MinMax1/2  "gamma min D"
  Discrete Gamma Measurement (D bridge)/2 -> Sum1/2
  Discrete Gamma Measurement (D bridge)/3 -> Terminator2/1
  Discrete Gamma Measurement (Y bridge)/2 -> Sum1/1
  Discrete Gamma Measurement (Y bridge)/3 -> Selector/1
  Discrete Gamma Measurement (Y bridge)/1 -> MinMax1/1  "gamma min Y"
  Vabc/1 -> Discrete Gamma Measurement (D bridge)/2, Discrete Gamma Measurement (Y bridge)/2

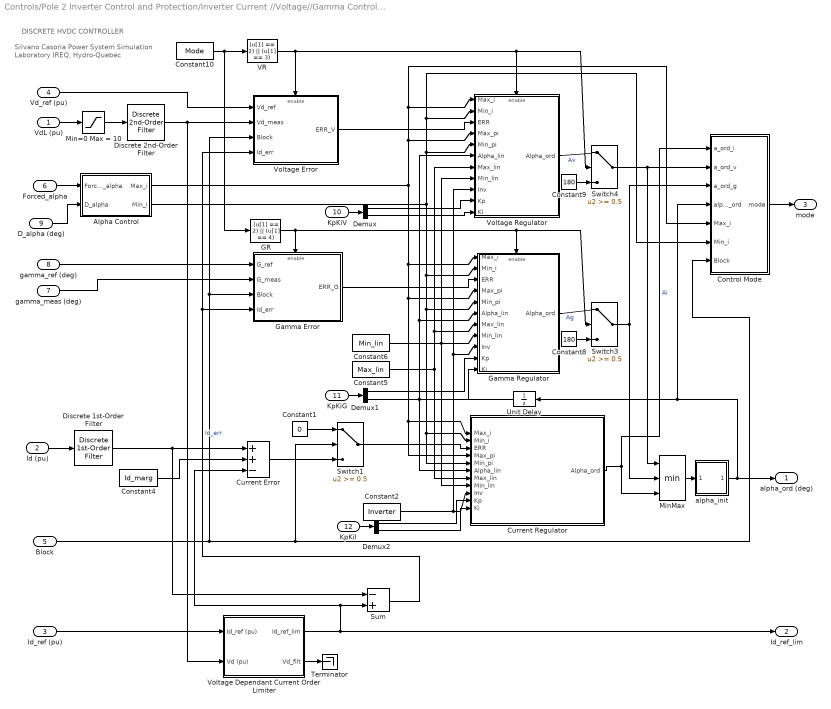
== system Controls/Pole 2 Inverter Control and Protection/Inverter Current //Voltage//Gamma Controller  ==
  note: Silvano Casoria
      | Power System Simulation Laboratory
      |  IREQ, Hydro-Quebec
  note: DISCRETE HVDC CONTROLLER
  VdL (pu) : Inport
  Id (pu) : Inport  Port=2
  Id_ref (pu) : Inport  Port=3
  Vd_ref (pu) : Inport  Port=4
  Block : Inport  Port=5
  Forced_alpha : Inport  Port=6
  gamma_meas (deg) : Inport  Port=7
  gamma_ref (deg) : Inport  Port=8
  D_alpha (deg) : Inport  Port=9
  KpKiV : Inport  Port=10
  KpKiG : Inport  Port=11
  KpKiI : Inport  Port=12
  Alpha Control : Subsystem
  Constant1 : Constant  Value=0
  Constant10 : Constant  Value=Mode
  Constant2 : Constant  Value=Inverter
  Constant4 : Constant  Value=Id_marg
  Constant5 : Constant  Value=Max_lin
  Constant6 : Constant  Value=Min_lin
  Constant8 : Constant  Value=180
  Constant9 : Constant  Value=180
  "Control Mode " : Subsystem
  Current Error : Sum  Inputs=++-  InputSameDT=on  SaturateOnIntegerOverflow=on  OutDataTypeStr=Inherit: Same as first input
  Current Regulator : Subsystem  mask(PI Regulator  With  External  Limits (Discrete)){Kp=Kp_I, Ki=Ki_I, IC_i=ICi_I, On_lin=on, dt=dt}
      mask prompts: Kp "Kp (deg/pu):"; Ki "Ki (deg/pu/s):"; IC_i "Integrator Initial Condition (deg):"; On_lin "Linearization  (On)"; dt "Sample time (s):"
      mask help: For the linearization it is important to specifie the mode of operation i.e. rectifier or inverter (negation of rectifier).
      mask Display: disp('PI Regulator\nWith external limits\n(Linearized Kp)\n(Discrete)\n\n')
  Demux : Demux  Outputs=2
  Demux1 : Demux  Outputs=2
  Demux2 : Demux  Outputs=2
  Discrete 1st-Order Filter : powerlib_extras/Discrete  Control Blocks/Discrete 1st-Order Filter  FilterType=Lowpass  Tc=T_I  Ts=dt  Initialize=off  Vac_Init=[0.8 -25 60]  Vdc_Init=-0.4  PlotResponse=off  param1=[1 500 0.1]
  Discrete 2nd-Order Filter : powerlib_extras/Discrete  Control Blocks/Discrete  2nd-Order Filter  FilterType=Lowpass  Fo=f0_V  Zeta=Z_V  Ts=dt  Initialize=off  Vac_Init=[0.8 -25 60]  Vdc_Init=-0.4  PlotResponse=off  param1=[1 500 1]
  GR : Fcn  Expr=(u[1] == 2) || (u[1] == 4)
  Gamma Error : Subsystem  TreatAsAtomicUnit=on
  Gamma Regulator : Subsystem  TreatAsAtomicUnit=on
  Min=0 Max = 10 : Saturate  UpperLimit=10  LowerLimit=0
  MinMax : MinMax  Inputs=3  InputSameDT=on  SaturateOnIntegerOverflow=on
  Sum : Sum  Inputs=-+  InputSameDT=on  SaturateOnIntegerOverflow=on  OutDataTypeStr=Inherit: Same as first input
  Switch1 : Switch  Threshold=0.5
  Switch3 : Switch  Threshold=0.5
  Switch4 : Switch  Threshold=0.5
  Terminator : Terminator
  Unit Delay : UnitDelay  SampleTime=dt  HasFrameUpgradeWarning=on
  VR : Fcn  Expr=(u[1] == 2) || (u[1] == 3)
  Voltage Dependant Current Order Limiter : Subsystem  mask(Voltage Dependent Current Order Limiter  (Discrete)){Vd_seuil=Vd_seuil, Vd_min=Vd_min, Id_min=Id_min, Id_min_abs=Id_min_abs, Tu=Tup, pas=dt}
      mask prompts: Vd_seuil "Vd seuil (pu):"; Vd_min "Vd min (pu):"; Id_min "Id min (pu):"; Id_min_abs "Id min abs (pu):"; Tu "Up Time constant (s):"; pas "Sample time (s):"
      mask Display: disp('VDCOL\n (Discrete)')
  Voltage Error : Subsystem  TreatAsAtomicUnit=on
  Voltage Regulator : Subsystem  TreatAsAtomicUnit=on
  alpha_init : Subsystem
  alpha_ord (deg) : Outport
  Id_ref_lim : Outport  Port=2
  mode : Outport  Port=3
  wires:
  Demux2/1 -> Current Regulator/10(Kp)
  Demux2/2 -> Current Regulator/11(Ki)
  KpKiI/1 -> Demux2/1
  Demux1/1 -> Gamma Regulator/10(Kp)
  Demux1/2 -> Gamma Regulator/11(Ki)
  KpKiG/1 -> Demux1/1
  Demux/1 -> Voltage Regulator/10(Kp)
  Demux/2 -> Voltage Regulator/11(Ki)
  KpKiV/1 -> Demux/1
  Forced_alpha/1 -> Alpha Control/1(Forced_alpha)
  "Control Mode "/1(mode) -> mode/1
  Voltage Error/1(ERR_V) -> Voltage Regulator/3(ERR)
  Vd_ref (pu)/1 -> Voltage Error/1(Vd_ref)
  Sum/1 -> Gamma Error/4(Id_err), Voltage Error/4(Id_err)  "Id_err"
  gamma_meas (deg)/1 -> Gamma Error/2(G_meas)
  gamma_ref (deg)/1 -> Gamma Error/1(G_ref)
  Gamma Error/1(ERR_G) -> Gamma Regulator/3(ERR)
  Constant1/1 -> Switch1/1
  Switch4/1 -> "Control Mode "/2(a_ord_v), MinMax/1
  Switch3/1 -> "Control Mode "/3(a_ord_g), MinMax/2
  Current Regulator/1(Alpha_ord) -> "Control Mode "/1("a_ord_i "), MinMax/3  "Ai"
  Constant9/1 -> Switch4/3
  Voltage Regulator/1(Alpha_ord) -> Switch4/1  "Av"
  Constant8/1 -> Switch3/3
  Gamma Regulator/1(Alpha_ord) -> Switch3/1  "Ag"
  Switch1/1 -> Current Regulator/3(ERR)
  Constant2/1 -> Current Regulator/9(Inv), Gamma Regulator/9(Inv), Voltage Regulator/9(Inv)
  Block/1 -> Voltage Error/3(Block), Gamma Error/3(Block), "Control Mode "/7(Block), Switch1/2
  Alpha Control/2(Min_i) -> Voltage Regulator/5(Min_pi), "Control Mode "/6(Min_i), Voltage Regulator/2(Min_i), Gamma Regulator/2(Min_i), Gamma Regulator/5(Min_pi), Current Regulator/2(Min_i), Current Regulator/5(Min_pi)
  Constant5/1 -> Current Regulator/7(Max_lin), Voltage Regulator/7(Max_lin), Gamma Regulator/7(Max_lin)
  alpha_init/1(Out1) -> "Control Mode "/4(alpha_ord), Unit Delay/1, alpha_ord (deg)/1
  Unit Delay/1 -> Current Regulator/6(Alpha_lin), Voltage Regulator/6(Alpha_lin), Gamma Regulator/6(Alpha_lin)
  MinMax/1 -> alpha_init/1(In1)
  Current Error/1 -> Switch1/3
  Discrete 1st-Order Filter/1 -> Current Error/1, Sum/1
  Id (pu)/1 -> Discrete 1st-Order Filter/1
  VdL (pu)/1 -> Min=0 Max = 10/1
  Min=0 Max = 10/1 -> Discrete 2nd-Order Filter/1
  Discrete 2nd-Order Filter/1 -> Voltage Error/2(Vd_meas), Voltage Dependant Current Order Limiter/2(Vd (pu))
  Voltage Dependant Current Order Limiter/1(Id_ref_lim) -> Current Error/3, Sum/2, Id_ref_lim/1
  Voltage Dependant Current Order Limiter/2(Vd_filt) -> Terminator/1
  Id_ref (pu)/1 -> Voltage Dependant Current Order Limiter/1(Id_ref (pu))
  Constant4/1 -> Current Error/2
  Constant6/1 -> Current Regulator/8(Min_lin), Voltage Regulator/8(Min_lin), Gamma Regulator/8(Min_lin)
  Alpha Control/1(Max_i) -> Voltage Regulator/4(Max_pi), "Control Mode "/5(Max_i), Voltage Regulator/1(Max_i), Gamma Regulator/1(Max_i), Gamma Regulator/4(Max_pi), Current Regulator/1(Max_i), Current Regulator/4(Max_pi)
  D_alpha (deg)/1 -> Alpha Control/2(D_alpha)
  VR/1 -> Voltage Regulator/Enable, Switch4/2, Voltage Error/Enable
  Constant10/1 -> GR/1, VR/1
  GR/1 -> Gamma Regulator/Enable, Switch3/2, Gamma Error/Enable

== system Controls/Pole 2 Inverter Control and Protection/Inverter Protections ==
  Uabc (pu) : Inport
  1st-Order T=3.3 ms : powerlib_extras/Discrete  Control Blocks/Discrete 1st-Order Filter  FilterType=Lowpass  Tc=0.0033  Ts=Tctrl  Initialize=off  Vac_Init=[0.8 -25 60]  Vdc_Init=-0.4  PlotResponse=off  param1=[1 500 0.1]
  Commutation Failure Prevention Control (CFPREV) : Subsystem  mask(Commutation Failure Prevention Control){STATE=on, T_ss=0.64, ab_level=0.1, ab_gain=25, z_level=0.1, z_gain=25, fn=60, Filter=[2.0, 1.0], Ts=Tctrl}
      mask prompts: STATE "ON State"; T_ss "Simulation Steady_State Time (s):"; ab_level "ab level (pu):"; ab_gain "ab gain (deg/pu):"; z_level "z level (pu):"; z_gain "z gain (deg/pu):"; fn "Base frequency (Hz):"; Filter "Filter Time const. and Iinitial condition [T(s), Ic (pu)]:"; Ts "Sample Time (s):"
      mask help:
      | The protective function, used in the inverter, mitigates commutation failures due to AC voltage dips. After a fault detection (three-phase or one-phase) an angle value (AMIN_CFPREV) is sent to the converter control in order to be deducted from the maximum delay angle limit (alpha_max). Practicaly, the commutation margin is consequently enlarged reducing therfore the risk of commutation failures.
      |
      |      The CLARK transformation is used for three-phase fault  detection and the zero-sequence voltage evaluation. The detection is based  on instantaneous values, which ensure fast reaction of the control system when AC faults occurs.
      |
      |      Press Help to get the reference with the  detailed description of the function and  parameters.
      |
      | Note: To accelerate the function initialisation, the first parameter (Simulation Steady_State Time) is used. It corresponds to the time when the input voltages reache  the steady-state value.
      mask init:
      | T_periode = 0.6/fn;    % More then half the period
      | filt_tc = Filter(1);
      | filt_ic = Filter(2);
      | 
      | if (STATE)
      | 	str = 'ON';
      | else
      | 	str = 'OFF';
      | end
      mask Help:
      | Ref. "A Novel Method to Mitigate Commutation Failures in HVDC Systems,"
      | Lidong Zhang, Lars Dofnas ABB Utilities Power System Technology,
      | Proceedings PowerCon 2002, Volume: 1 , 13-17 Oct. 2002,  Page(s): 51-56 vol.1.
      mask Display: disp(['\n\n\n State:[',str,']'])
  Informations : Subsystem
      mask Display: disp('?')
  Low AC Voltage Detection (LACVD) : Subsystem  TreatAsAtomicUnit=on  mask(Low AC voltage detection){STATE=on, Ref_1=0.75, dt=Ts}
      mask prompts: STATE "ON State"; Ref_1 "Detection level (pu):"; dt "Sample time (s):"
      mask help:
      | This bloc detects a low AC voltage condition on the commutation busbar and is used in the DC protection scheme. Its purpose is to descriminate between a drop in the AC voltage caused by a fault on the DC line or by a fault on the AC side.
      |
      |      An AC fault detection (Low_ac_voltage output signal) will occur when the AC voltage input (recified three-phase AC voltage) drops below a certain reference value (Detection
      | level).
      |
      |      In order to minimize the simulation time, an enabled susbystem having a sample time of 1 (ms) has been used in accordance with an acceptable precision.
      mask init:
      | if (STATE)
      | 	str = 'ON';
      | else
      | 	str = 'OFF';
      | end
      mask Display: disp(['\n\n\n\nState:[',str,']'])
  Udio_6p : Subsystem
  Low_AC_Voltage : Outport
  AMIN_CFPREV : Outport  Port=2
  wires:
  Commutation Failure Prevention Control (CFPREV)/1(AMIN_CFPREV (deg)) -> AMIN_CFPREV/1
  Low AC Voltage Detection (LACVD)/1(Low_AC_Voltage) -> Low_AC_Voltage/1
  Uabc (pu)/1 -> Udio_6p/1(Uabc (pu)), Commutation Failure Prevention Control (CFPREV)/1(Uabc (pu))
  Udio_6p/1(Udio_6p) -> 1st-Order T=3.3 ms/1
  1st-Order T=3.3 ms/1 -> Low AC Voltage Detection (LACVD)/1(Uac (pu))

== system Controls/Pole 2 Inverter Control and Protection/Polarity_check ==
  converter_position : Inport
  Vdc_line : Inport  Port=2
  Vdc_neutral : Inport  Port=3
  Idc_in : Inport  Port=4
  Add : Sum  Inputs=+-
  Constant : Constant
  Constant1 : Constant  Value=-1
  Constant2 : Constant  Value=3
  Discrete 1st-Order Filter : powerlib_extras/Discrete  Control Blocks/Discrete 1st-Order Filter  FilterType=Lowpass  Tc=5  Ts=Tctrl  Initialize=off  Vac_Init=[0.8 -25 60]  Vdc_Init=-0.4  PlotResponse=off  param1=[1 500 0.1]
  MinMax : MinMax  Function=max  SampleTime=Tctrl
  Multiport Switch : MultiPortSwitch  DataPortOrder=Zero-based contiguous  Inputs=2  zeroidx=on  SaturateOnIntegerOverflow=off  InputSameDT=off
  Mux : Mux  Inputs=2
  Product : Product  RndMeth=Zero
  Product1 : Product  RndMeth=Zero
  Product2 : Product  RndMeth=Zero
  Relational Operator : RelationalOperator  OutDataTypeStr=boolean  InputSameDT=off
  Vdc_meas : Outport
  Idc_meas : Outport  Port=2
  wires:
  Product2/1 -> Idc_meas/1
  Relational Operator/1 -> Multiport Switch/1
  Constant2/1 -> Relational Operator/2
  converter_position/1 -> Relational Operator/1
  Idc_in/1 -> Product2/2
  Multiport Switch/1 -> Product2/1, Product1/1, Product/1
  Constant1/1 -> Multiport Switch/3
  Constant/1 -> Multiport Switch/2
  Vdc_neutral/1 -> Product1/2
  Product1/1 -> Discrete 1st-Order Filter/1
  Product/1 -> Mux/1, Add/1
  Vdc_line/1 -> Product/2
  MinMax/1 -> Vdc_meas/1
  Mux/1 -> MinMax/1
  Add/1 -> Mux/2
  Discrete 1st-Order Filter/1 -> Add/2

== system Controls/Pole 2 Inverter Control and Protection/Ref_and_step_ctrl ==
  Vd_step : Inport
  Gamma_step : Inport  Port=2
  Add : Sum
  Add1 : Sum
  Discrete Monostable1 : powerlib_extras/Discrete  Control Blocks/Discrete Monostable  EdgeDetect=Rising  t_mono=0.2  ic=0  Ts=Tctrl
  Discrete Monostable2 : powerlib_extras/Discrete  Control Blocks/Discrete Monostable  EdgeDetect=Rising  t_mono=0.1  ic=0  Ts=Tctrl
  Gamma min : Constant  Value=18
  Vd_ref : Constant  Value=1.0
  g : Gain  Gain=5  SaturateOnIntegerOverflow=on  OutDataTypeStr=Inherit: Same as input  ParamDataTypeStr=Inherit: Same as input
  g1 : Gain  Gain=-0.1  SaturateOnIntegerOverflow=on  OutDataTypeStr=Inherit: Same as input  ParamDataTypeStr=Inherit: Same as input
  Vd_ref_out : Outport
  Gamma_ref_out : Outport  Port=2
  wires:
  Add/1 -> Gamma_ref_out/1
  Gamma_step/1 -> Discrete Monostable1/1
  Discrete Monostable1/1 -> g/1
  Gamma min/1 -> Add/2
  g/1 -> Add/1
  Vd_step/1 -> Discrete Monostable2/1
  Add1/1 -> Vd_ref_out/1
  g1/1 -> Add1/1
  Discrete Monostable2/1 -> g1/1
  Vd_ref/1 -> Add1/2

== system Controls/Pole 2 Rectifier Control and Protection/12-pulse Firing Control ==
  alpha_ord (deg) : Inport
  Vabc (pu) : Inport  Port=2
  Block : Inport  Port=3
  Data Type Conversion : DataTypeConversion  OutDataTypeStr=double
  Mux2 : Mux  Inputs=6
  PLL : Subsystem
  Freq : Outport
  fpuR : Outport  Port=2
  wires:
  Data Type Conversion/1 -> Mux2/6
  Mux2/1 -> fpuR/1
  Block/1 -> Data Type Conversion/1
  alpha_ord (deg)/1 -> Mux2/1
  PLL/4(Freq) -> Mux2/5, Freq/1
  PLL/3(Vc) -> Mux2/4
  PLL/2(Vb) -> Mux2/3
  PLL/1(Va) -> Mux2/2
  Vabc (pu)/1 -> PLL/1(Vabc(pu))
